simulink model "current_ctl_loop_task_Harness2"  (R2023a)
settings: configuration reference "config" (kept outside this file)
libraries: servo_hub_lib x1
settings Model: DataDictionary=model_config.sldd  Creator=hcch1  LastModifiedBy=hcch1
settings ConfigSetRef: SourceName=config

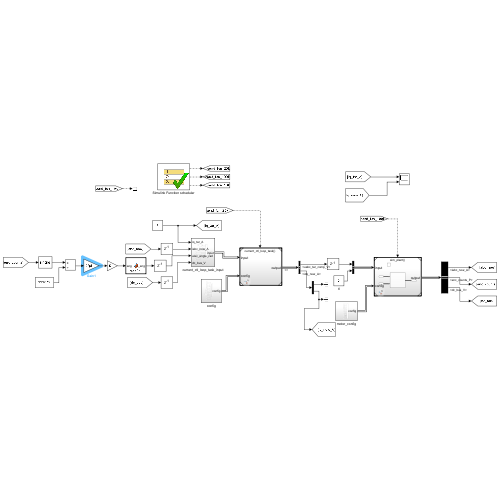
[thumbnail: Simulink's stored preview of the top-level diagram]
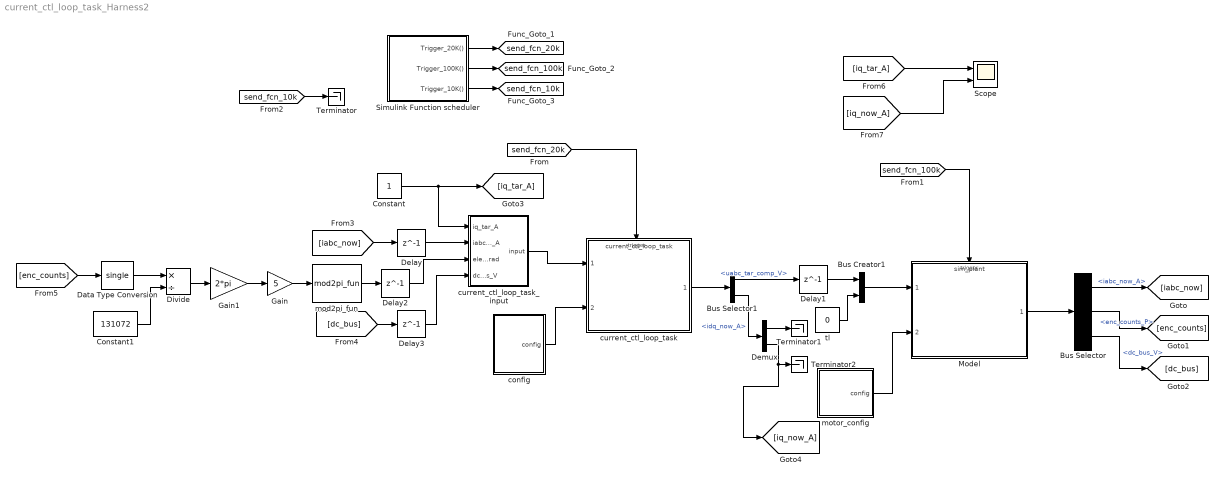
== system current_ctl_loop_task_Harness2 ==
  Bus Creator1 : BusCreator  Inputs=2  OutDataTypeStr=Bus: SimPlantInput  NonVirtualBus=on
      settings: InheritFromInputs=off
  Bus Selector : BusSelector  OutputSignals=iabc_now_A,enc_counts_P,dc_bus_V
  Bus Selector1 : BusSelector  OutputSignals=uabc_tar_comp_V,idq_now_A
  Constant : Constant  OutDataTypeStr=single
  Constant1 : Constant  Value=131072  OutDataTypeStr=single
  Data Type Conversion : DataTypeConversion  OutDataTypeStr=single  SaturateOnIntegerOverflow=off  RndMeth=Floor
  Delay{,1..3} (4 alike) : Delay  DelayLength=1
  Demux : Demux  Outputs=2
  Divide : Product  Inputs=*/
  Gain : Gain  Gain=5
  Gain1 : Gain  Gain=2*pi
  Model : ModelReference  ModelNameDialog=sim_plant.slx  SimulationMode=Normal  ModelReferenceVersion=1.108  TriggerPortName=Trigger  TriggerPortTriggerType=function-call  TriggerPortStatesWhenEnabling=held
  Scope : Scope  NumInputPorts=2
  Simulink Function scheduler : Test Sequence  Tag=__SLT_FCN_CALL__  TreatAsAtomicUnit=on
  Terminator : Terminator
  Terminator1 : Terminator
  Terminator2 : Terminator
  config : Subsystem
  current_ctl_loop_task : ModelReference  ModelNameDialog=current_ctl_loop_task  SimulationMode=Normal  ModelReferenceVersion=2.1046  TriggerPortName=Trigger  TriggerPortTriggerType=function-call  TriggerPortStatesWhenEnabling=held
  current_ctl_loop_task_input : Subsystem
  mod2pi_fun : servo_hub_lib/fast_math/mod2pi_fun  SystemSampleTime=-1  VariantActivationTime=update diagram  Latency=0  AutoFrameSizeCalculation=off
      settings: LibrarySourceBlock=|
      | simulink/User-Defined
      | Functions/MATLAB Function
  motor_config : Subsystem
  tl : Constant  Value=0  OutDataTypeStr=single
  tag scope: send_fcn_100k=global, send_fcn_10k=global, send_fcn_20k=global
  wires:
  Simulink Function scheduler/2(Trigger_100K()) -> [send_fcn_100k]
  Simulink Function scheduler/3(Trigger_10K()) -> [send_fcn_10k]
  Simulink Function scheduler/1(Trigger_20K()) -> [send_fcn_20k]
  [send_fcn_20k] -> current_ctl_loop_task/Trigger
  [send_fcn_100k] -> Model/Trigger
  [send_fcn_10k] -> Terminator/1
  config/1(config) -> current_ctl_loop_task/2
  current_ctl_loop_task_input/1(input) -> current_ctl_loop_task/1
  Constant/1 -> [iq_tar_A], current_ctl_loop_task_input/1(iq_tar_A)
  Bus Selector/1 -> [iabc_now]  "<iabc_now_A>"
  Bus Selector/2 -> [enc_counts]  "<enc_counts_P>"
  Bus Selector/3 -> [dc_bus]  "<dc_bus_V>"
  [iabc_now] -> Delay/1
  [dc_bus] -> Delay3/1
  motor_config/1(config) -> Model/2
  [enc_counts] -> Data Type Conversion/1
  Constant1/1 -> Divide/2
  Data Type Conversion/1 -> Divide/1
  Divide/1 -> Gain1/1
  Gain/1 -> mod2pi_fun/1
  mod2pi_fun/1 -> Delay2/1
  current_ctl_loop_task/1 -> Bus Selector1/1
  Bus Selector1/1 -> Delay1/1  "<uabc_tar_comp_V>"
  Bus Creator1/1 -> Model/1
  tl/1 -> Bus Creator1/2
  Bus Selector1/2 -> Demux/1  "<idq_now_A>"
  Demux/1 -> Terminator1/1
  Demux/2 -> [iq_now_A], Terminator2/1
  Delay1/1 -> Bus Creator1/1
  [iq_tar_A] -> Scope/1
  [iq_now_A] -> Scope/2
  Model/1 -> Bus Selector/1
  Delay/1 -> current_ctl_loop_task_input/2(iabc_now_A)
  Delay2/1 -> current_ctl_loop_task_input/3(elec_angle_rad)
  Delay3/1 -> current_ctl_loop_task_input/4(dc_bus_V)
  Gain1/1 -> Gain/1

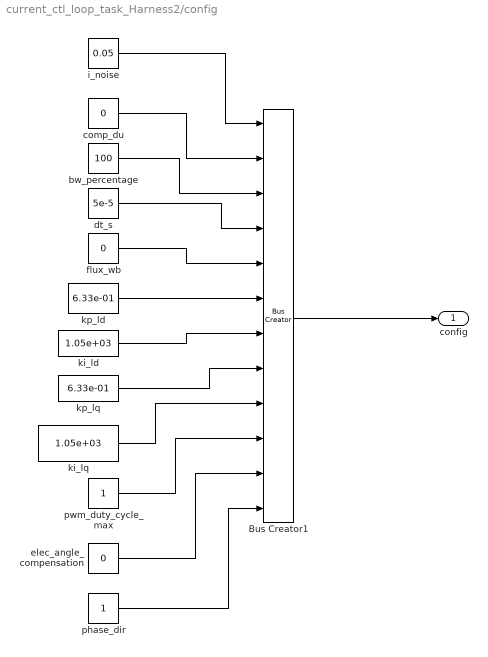
== system current_ctl_loop_task_Harness2/config ==
  Bus Creator1 : BusCreator  Inputs=12  OutDataTypeStr=Bus: CurrentCtlConfig  NonVirtualBus=on
      settings: InheritFromInputs=off
  bw_percentage : Constant  Value=100  OutDataTypeStr=single
  comp_du : Constant  Value=0  OutDataTypeStr=single
  dt_s : Constant  Value=5e-5  OutDataTypeStr=single
  elec_angle_compensation : Constant  Value=0  OutDataTypeStr=single
  flux_wb : Constant  Value=0  OutDataTypeStr=single
  i_noise : Constant  Value=0.05  OutDataTypeStr=single
  ki_ld : Constant  Value=1.05e+03  OutDataTypeStr=single
  ki_lq : Constant  Value=1.05e+03  OutDataTypeStr=single
  kp_ld : Constant  Value=6.33e-01  OutDataTypeStr=single
  kp_lq : Constant  Value=6.33e-01  OutDataTypeStr=single
  phase_dir : Constant  OutDataTypeStr=int8  LockScale=on
  pwm_duty_cycle_max : Constant  OutDataTypeStr=single
  config : Outport
  wires:
  flux_wb/1 -> Bus Creator1/5
  pwm_duty_cycle_max/1 -> Bus Creator1/10
  comp_du/1 -> Bus Creator1/2
  bw_percentage/1 -> Bus Creator1/3
  elec_angle_compensation/1 -> Bus Creator1/11
  i_noise/1 -> Bus Creator1/1
  Bus Creator1/1 -> config/1
  kp_lq/1 -> Bus Creator1/8
  ki_ld/1 -> Bus Creator1/7
  phase_dir/1 -> Bus Creator1/12
  kp_ld/1 -> Bus Creator1/6
  ki_lq/1 -> Bus Creator1/9
  dt_s/1 -> Bus Creator1/4

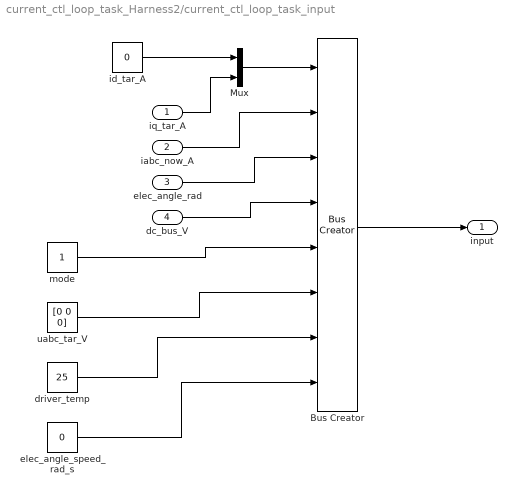
== system current_ctl_loop_task_Harness2/current_ctl_loop_task_input ==
  iq_tar_A : Inport
  iabc_now_A : Inport  Port=2
  elec_angle_rad : Inport  Port=3
  dc_bus_V : Inport  Port=4
  Bus Creator : BusCreator  Inputs=8  OutDataTypeStr=Bus: CurrentCtlInput  NonVirtualBus=on
      settings: InheritFromInputs=off
  Mux : Mux  Inputs=2
  driver_temp : Constant  Value=25  OutDataTypeStr=single  SampleTime=-1
  elec_angle_speed_rad_s : Constant  Value=0  OutDataTypeStr=single  SampleTime=-1
  id_tar_A : Constant  Value=0  OutDataTypeStr=single  SampleTime=-1
  mode : Constant  OutDataTypeStr=uint8  SampleTime=-1
  uabc_tar_V : Constant  Value=[0 0 0]  OutDataTypeStr=single  SampleTime=-1
  input : Outport
  wires:
  Mux/1 -> Bus Creator/1
  Bus Creator/1 -> input/1
  dc_bus_V/1 -> Bus Creator/4
  iabc_now_A/1 -> Bus Creator/2
  elec_angle_rad/1 -> Bus Creator/3
  iq_tar_A/1 -> Mux/2
  id_tar_A/1 -> Mux/1
  mode/1 -> Bus Creator/5
  uabc_tar_V/1 -> Bus Creator/6
  driver_temp/1 -> Bus Creator/7
  elec_angle_speed_rad_s/1 -> Bus Creator/8

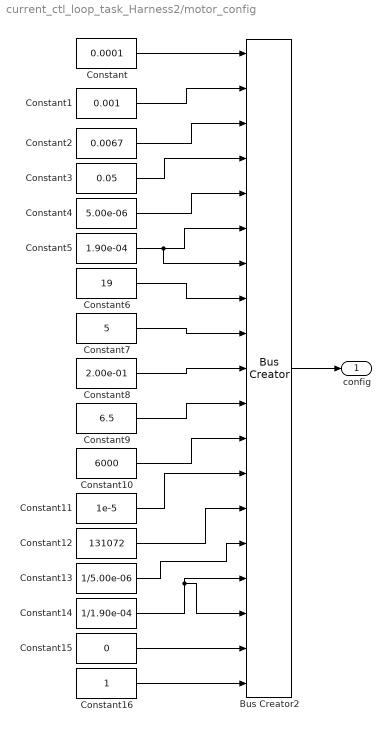
== system current_ctl_loop_task_Harness2/motor_config ==
  Bus Creator2 : BusCreator  Inputs=19  OutDataTypeStr=Bus: SimPlantConfig  NonVirtualBus=on
      settings: InheritFromInputs=off
  Constant : Constant  Value=0.0001  OutDataTypeStr=single
  Constant1 : Constant  Value=0.001  OutDataTypeStr=single
  Constant10 : Constant  Value=6000  OutDataTypeStr=single
  Constant11 : Constant  Value=1e-5  OutDataTypeStr=single
  Constant12 : Constant  Value=131072  OutDataTypeStr=uint32
  Constant13 : Constant  Value=1/5.00e-06  OutDataTypeStr=single
  Constant14 : Constant  Value=1/1.90e-04  OutDataTypeStr=single
  Constant15 : Constant  Value=0  OutDataTypeStr=int64
  Constant16 : Constant  OutDataTypeStr=single
  Constant2 : Constant  Value=0.0067  OutDataTypeStr=single
  Constant3 : Constant  Value=0.05  OutDataTypeStr=single
  Constant4 : Constant  Value=5.00e-06  OutDataTypeStr=single
  Constant5 : Constant  Value=1.90e-04  OutDataTypeStr=single
  Constant6 : Constant  Value=19  OutDataTypeStr=single
  Constant7 : Constant  Value=5  OutDataTypeStr=single
  Constant8 : Constant  Value=2.00e-01  OutDataTypeStr=single
  Constant9 : Constant  Value=6.5  OutDataTypeStr=single
  config : Outport
  wires:
  Bus Creator2/1 -> config/1
  Constant/1 -> Bus Creator2/1
  Constant1/1 -> Bus Creator2/2
  Constant2/1 -> Bus Creator2/3
  Constant3/1 -> Bus Creator2/4
  Constant4/1 -> Bus Creator2/5
  Constant5/1 -> Bus Creator2/6, Bus Creator2/7
  Constant6/1 -> Bus Creator2/8
  Constant7/1 -> Bus Creator2/9
  Constant8/1 -> Bus Creator2/10
  Constant9/1 -> Bus Creator2/11
  Constant10/1 -> Bus Creator2/12
  Constant11/1 -> Bus Creator2/13
  Constant12/1 -> Bus Creator2/14
  Constant13/1 -> Bus Creator2/15
  Constant14/1 -> Bus Creator2/17, Bus Creator2/16
  Constant15/1 -> Bus Creator2/18
  Constant16/1 -> Bus Creator2/19

== stateflow chart current_ctl_loop_task_Harness2/Simulink Function scheduler ==
  settings: updateMethod=DISCRETE  sampleTime=1.0E-5
  state Run
    num = 0;
    pos_num = 0;
    send(Trigger_10K);
    send(Trigger_20K);
    send(Trigger_100K);
  state step_1
    num = num +1;
    pos_num = pos_num+1;
    if (num >= 5)
    send(Trigger_20K);
    num  = 0;
    end
    if (pos_num>= 10)
    send(Trigger_10K);
    pos_num= 0;
    end
    send(Trigger_100K);
    settings: description="产生100k  20k  10k 函数周期调用"
  (default) -> Run
  Run -> step_1 : [
      | true
      | ]
  step_1 -> Run : [
      | false
      | ]
  data: num local; pos_num local
  events: Trigger_20K output FUNCTION_CALL_EVENT; Trigger_100K output FUNCTION_CALL_EVENT; Trigger_10K output FUNCTION_CALL_EVENT
